simulink model "Adaptive_Event_send"  (R2023b)
settings: Solver=FixedStepDiscrete  StartTime=0.0  StopTime=50  RelTol=1e-3  EnableMultiTasking=on
undefined symbols (not defined in the file): gray, Rec, SDTV
libraries: visiontextngfix x4, visionconversions x3, visiongeotforms x2, autosarlibaprouting x1, raspberrypiAVlib x1
settings Model: Creator=seame-workstation09  LastModifiedBy=seame-workstation09
settings SolverCC: PositivePriorityOrder=on
settings OptimizationCC: DefaultParameterBehavior=Inlined  UseDivisionForNetSlopeComputation=on  GainParamInheritBuiltInType=on  UseFloatMulNetSlope=on  EnhancedBackFolding=on  PassReuseOutputArgsAs=Individual arguments  ZeroExternalMemoryAtStartup=off  ZeroInternalMemoryAtStartup=off  NoFixptDivByZeroProtection=on  EfficientFloat2IntCast=on  MaxStackSize=64  OptimizeBlockOrder=speed  DifferentSizesBufferReuse=on  OptimizationCustomize=off  EfficientTunableParamExpr=on
settings DebuggingCC: ParameterTunabilityLossMsg=error
settings HardwareCC: ProdBitPerLong=64  ProdLargestAtomicInteger=LongLong  ProdLargestAtomicFloat=Double  ProdLongLongMode=on  ProdHWDeviceType=ARM Compatible->ARM 64-bit (LP64)
settings SFSimCC: SimGenImportedTypeDefs=on  MATLABDynamicMemAlloc=off  SimTargetLang=C++
settings RTWCC: Description=AUTOSAR Adaptive  SystemTargetFile=autosar_adaptive.tlc  HardwareBoard=Embedded Coder Linux Docker Container  GenCodeOnly=on  TemplateMakefile=ert_default_tmf  Toolchain=AUTOSAR Adaptive Linux Executable  BuildConfiguration=Faster Runs  DataTypeReplacement=CDataTypesFixedWidth  TargetLang=C++
settings CodeAppCC: ForceParamTrailComments=on  IgnoreCustomStorageClasses=off  MaxIdLength=63  OperatorAnnotations=on  SimulinkDataObjDesc=on  SFDataObjDesc=on  CustomSymbolStrGlobalVar=rt$N$M  CustomSymbolStrType=$N$M  CustomSymbolStrFcn=$N$M$F  CustomSymbolStrMacro=$N$M  InsertBlockDesc=on
settings AUTOSARAdaptiveTargetCC: TargetFcnLib=ansi_tfl_table_tmw.mat  GenFloatMathFcnCalls=NOT IN USE  TargetLangStandard=C++11 (ISO)  CodeReplacementLibrary=None  UtilityFuncGeneration=Auto  MultiwordTypeDef=System defined  MultiwordLength=2048  DynamicStringBufferSize=256  GenerateFullHeader=on  InferredTypesCompatibility=off  GenerateSampleERTMain=off  GenerateTestInterfaces=off  ModelReferenceCompliant=on  ParMdlRefBuildCompliant=on  CompOptLevelCompliant=on  ConcurrentExecutionCompliant=on  IncludeMdlTerminateFcn=on  CombineOutputUpdateFcns=on  CombineSignalStateStructs=off  GroupInternalDataByFunction=off  SuppressErrorStatus=on  IncludeFileDelimiter=Auto  ERTCustomFileBanners=off  SupportAbsoluteTime=on  LogVarNameModifier=rt_  MatFileLogging=off  CodeInterfacePackaging=C++ class  PurelyIntegerCode=off  SupportNonFinite=off  SupportComplex=on  SupportContinuousTime=off  SupportNonInlinedSFcns=off  RemoveDisableFunc=off  RemoveResetFunc=on  SupportVariableSizeSignals=off  ParenthesesLevel=Nominal  CastingMode=Nominal  MATLABClassNameForMDSCustomization=Simulink.SoftwareTarget.TargetSpecificTriggerConfigurationBase  ModelStepFunctionPrototypeControlCompliant=off  CPPClassGenCompliant=on  AutosarCompliant=on  MDXCompliant=off  GRTInterface=off  GenerateAllocFcn=off  UseToolchainInfoCompliant=on  GenerateSharedConstants=on  CoderGroups=[]  AccessMethods=[]  LookupTableObjectStructAxisOrder=2,1,3,4,...  LUTObjectStructOrderExplicitValues=Size,Breakpoints,Table  LUTObjectStructOrderEvenSpacing=Size,Table,Breakpoints  ArrayLayout=Column-major  UnsupportedSFcnMsg=error  ERTHeaderFileRootName=$R$E  ERTSourceFileRootName=$R$E  ERTDataFileRootName=$R_data  OptimizeReductions=off  GenerateASAP2=off  DSAsUniqueAccess=off  ExtMode=on  ExtModeTransport=0  ExtModeStaticAlloc=off  ExtModeAutomaticAllocSize=on  ExtModeMaxTrigDuration=10  ExtModeStaticAllocSize=1000000  ExtModeTesting=off  ExtModeMexFile=ext_comm  ExtModeIntrfLevel=Level1  InlinedParameterPlacement=NonHierarchical  TargetOS=BareBoardExample  MultiInstanceErrorCode=Error  RootIOFormat=Structure reference  RTWCAPISignals=off  RTWCAPIParams=off  RTWCAPIStates=off  RTWCAPIRootIO=off  ERTSrcFileBannerTemplate=ert_code_template.cgt  ERTHdrFileBannerTemplate=ert_code_template.cgt  ERTDataSrcFileTemplate=ert_code_template.cgt  ERTDataHdrFileTemplate=ert_code_template.cgt  ERTCustomFileTemplate=example_file_process.tlc  EnableDataOwnership=off  SignalDisplayLevel=10  ParamTuneLevel=10  GlobalDataDefinition=Auto  DataDefinitionFile=global.c  GlobalDataReference=Auto  ERTFilePackagingFormat=Modular  RateTransitionBlockCode=Inline  DataReferenceFile=global.h  PreserveExpressionOrder=off  PreserveIfCondition=off  ConvertIfToSwitch=on  PreserveExternInFcnDecls=on  PreserveStaticInFcnDecls=on  SuppressUnreachableDefaultCases=on  EnableSignedLeftShifts=on  EnableSignedRightShifts=on  ImplementImageWithCVMat=off  IndentStyle=K&R  IndentSize=2  NewlineStyle=Default  MaxLineWidth=80  EnableUserReplacementTypes=off  MaxIdInt64=INT64_MAX  MinIdInt64=INT64_MIN  MaxIdUint64=UINT64_MAX  MaxIdInt32=INT32_MAX  MinIdInt32=INT32_MIN  MaxIdUint32=UINT32_MAX  MaxIdInt16=INT16_MAX  MinIdInt16=INT16_MIN  MaxIdUint16=UINT16_MAX  MaxIdInt8=INT8_MAX  MinIdInt8=INT8_MIN  MaxIdUint8=UINT8_MAX  BooleanTrueId=true  BooleanFalseId=false  MemSecPackage=--- None ---  MemSecDataConstants=Default  MemSecDataIO=Default  MemSecDataInternal=Default  MemSecDataParameters=Default  MemSecFuncInitTerm=Default  MemSecFuncExecute=Default  MemSecFuncSharedUtil=Default  GroupConstants=Default  GroupRootInputs=Default  GroupRootOutputs=Default  GroupInternal=Default  GroupParameters=Default  GroupDataTransfer=Default  GroupSharedLocalDataStores=Default  GroupInstanceSpecificParameters=Default  GroupModelData=Default  ArrayContainerType=std::array  AutosarSchemaVersion=R21-11  AutosarMaxShortNameLength=128  AdaptiveAutosarXCPServerTransportLayer=XCPOnTCPIP  AdaptiveAutosarXCPServerTCPIPAddress=192.168.86.20  AdaptiveAutosarXCPServerPort=22  AdaptiveAutosarXCPServerVerbosity=off  AdaptiveAutosarUseCustomXCPServer=off

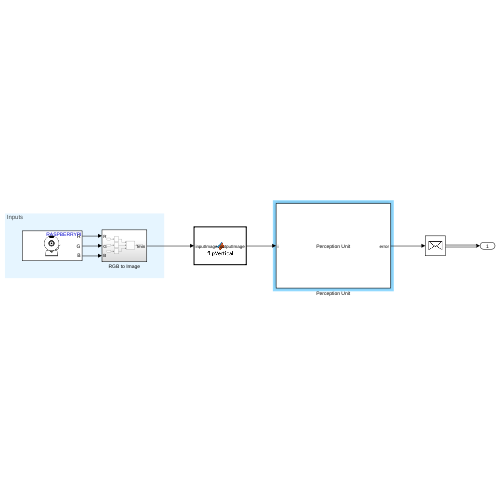
[thumbnail: Simulink's stored preview of the top-level diagram]
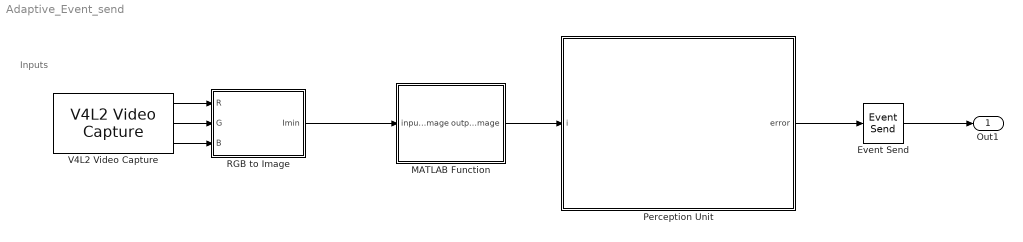
== system Adaptive_Event_send ==
  note: Inputs
  Event Send : autosarlibaprouting/Event Send
  MATLAB Function : MATLAB Function  TreatAsAtomicUnit=on
  Perception Unit : Subsystem  Description=Perception Unit
      mask Display: disp('Perception Unit');
  RGB to Image : Subsystem
  V4L2 Video Capture : raspberrypiAVlib/V4L2 Video Capture  DeviceName=/dev/video0  Resolution=640x480  CustomResolution=[2592,1944]  PixelFormat=RGB  SampleTime=0.1  pixelOrder=planar  simOutput=Colorbars  imSizeSelection=320x240  imSize=[640, 480]  roi=[0, 0, 640, 480]  m_devName='/dev/video0'  blockPlatform=LINUX  HorizontalFlip=off  VerticalFlip=off  Brightness=0.5  Saturation=0.5  Contrast=0.5  Sharpness=0.5  CameraPan=0  CameraTilt=0  CameraZoom=0.5  EnableManualFocus=on  ManualFocus=0.5
  Out1 : Outport
  wires:
  V4L2 Video Capture/1 -> RGB to Image/1(R)
  V4L2 Video Capture/2 -> RGB to Image/2(G)
  V4L2 Video Capture/3 -> RGB to Image/3(B)
  RGB to Image/1(Imin) -> MATLAB Function/1(inputImage)
  MATLAB Function/1(outputImage) -> Perception Unit/1(i)
  Perception Unit/1(error) -> Event Send/1
  Event Send/1 -> Out1/1

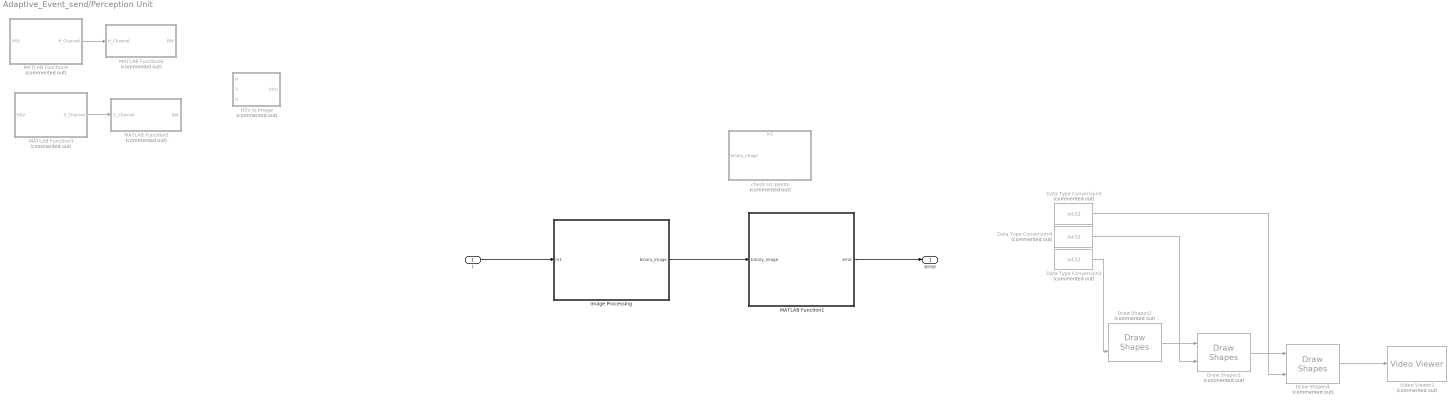
== system Adaptive_Event_send/Perception Unit ==
  i : Inport
  Data Type Conversion3 : DataTypeConversion  Commented=on  OutDataTypeStr=int32  SaturateOnIntegerOverflow=off  RndMeth=Floor
  Data Type Conversion4 : DataTypeConversion  Commented=on  OutDataTypeStr=int32  SaturateOnIntegerOverflow=off  RndMeth=Floor
  Data Type Conversion5 : DataTypeConversion  Commented=on  OutDataTypeStr=int32  SaturateOnIntegerOverflow=off  RndMeth=Floor
  Draw Shapes2 : visiontextngfix/Draw Shapes  Commented=on  shape=Rectangles  fill=off  lineWidth=1  fillClrSource=Specify via dialog  display=White  intensity=200  color=[0 255 0]  opacity=0.6  viewport=Entire image  antialiasing=off  inType=Obsolete  imagePorts=One multidimensional signal  roundingMode=Floor  overflowMode=off  memoryMode=Specify word length  memoryWordLength=16  prodOutputMode=Binary point scaling  prodOutputWordLength=32  prodOutputFracLength=14  memoryFracLength=15
  Draw Shapes3 : visiontextngfix/Draw Shapes  Commented=on  shape=Circles  fill=on  lineWidth=1  fillClrSource=Specify via dialog  display=Black  intensity=200  color=[0 255 0]  opacity=0.8  viewport=Entire image  antialiasing=off  inType=Obsolete  imagePorts=One multidimensional signal  roundingMode=Floor  overflowMode=off  memoryMode=Specify word length  memoryWordLength=16  prodOutputMode=Binary point scaling  prodOutputWordLength=32  prodOutputFracLength=14  memoryFracLength=15
  Draw Shapes4 : visiontextngfix/Draw Shapes  Commented=on  shape=Lines  fill=off  lineWidth=4  fillClrSource=Specify via dialog  display=Black  intensity=200  color=[255 0 0]  opacity=0.6  viewport=Entire image  antialiasing=off  inType=Obsolete  imagePorts=One multidimensional signal  roundingMode=Floor  overflowMode=off  memoryMode=Specify word length  memoryWordLength=16  prodOutputMode=Binary point scaling  prodOutputWordLength=32  prodOutputFracLength=14  memoryFracLength=14
  HSV to Image : Subsystem  Commented=on
  Image Processing : Subsystem
  MATLAB Function1 : MATLAB Function  TreatAsAtomicUnit=on
  MATLAB Function3 : MATLAB Function  Commented=on  TreatAsAtomicUnit=on
  MATLAB Function4 : MATLAB Function  Commented=on  TreatAsAtomicUnit=on
  MATLAB Function5 : MATLAB Function  Commented=on  TreatAsAtomicUnit=on
  MATLAB Function6 : MATLAB Function  Commented=on  TreatAsAtomicUnit=on
  Video Viewer2 : VideoViewer  Commented=on  colormapValue=gray(256)  FigPos=[498 952 1161 594]
  check src points : Subsystem  Commented=on
      settings: PortSchema="{\"entries\":[{\"content\":{\"sides\":[{\"content\":{\"connectorIds\":[\"In1\"]},\"type\":\"ConnectorPlacement.EquallySpacedRectSide\",\"uuid\":\"f9a6de61-1898-4465-aab1-5f75a88d6bc5\"},{\"content\":{\"side\":\"RIGHT\"},\"type\":\"ConnectorPlacement.EquallySpacedRectSide\",\"uuid\":\"22a87883-a793-424b-ac6e-07d139e6a826\"},{\"content\":{\"connectorIds\":[\"In2\"],\"side\":\"TOP\"},\"type\":\"ConnectorPlacement.EquallySpacedRectSide\",\"uuid\":\"93f3f8a5-f2dd-45b6-b00d-0d3a0a24e380\"}]},\"type\":\"ConnectorPlacement.EquallySpacedConnector\",\"uuid\":\"35037751-f37a-49b1-b87d-24865a03c27c\"}],\"packageUris\":[\"http://schema.mathworks.com/mf0/Connector/R2020b\"],\"version\":\"1.0\"}"
  error : Outport  VectorParamsAs1DForOutWhenUnconnected=off
  wires:
  MATLAB Function4/1(H_Channel) -> MATLAB Function6/1(H_Channel)
  MATLAB Function3/1(S_Channel) -> MATLAB Function5/1(S_Channel)
  i/1 -> Image Processing/1(In1)
  Image Processing/1(binary_image) -> MATLAB Function1/1(binary_image)
  Data Type Conversion3/1 -> Draw Shapes2/2
  Data Type Conversion4/1 -> Draw Shapes3/2
  Draw Shapes2/1 -> Draw Shapes3/1
  Draw Shapes3/1 -> Draw Shapes4/1
  Data Type Conversion5/1 -> Draw Shapes4/2
  MATLAB Function1/1(error) -> error/1
  Draw Shapes4/1 -> Video Viewer2/1

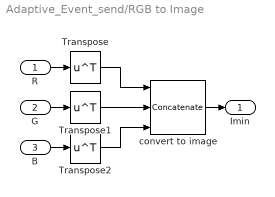
== system Adaptive_Event_send/RGB to Image ==
  R : Inport
  G : Inport  Port=2
  B : Inport  Port=3
  Transpose : Math  Operator=transpose
  Transpose1 : Math  Operator=transpose
  Transpose2 : Math  Operator=transpose
  convert to image : Concatenate  NumInputs=3  Mode=Multidimensional array  ConcatenateDimension=3
  Imin : Outport
  wires:
  R/1 -> Transpose/1
  G/1 -> Transpose1/1
  Transpose/1 -> convert to image/1
  Transpose1/1 -> convert to image/2
  B/1 -> Transpose2/1
  Transpose2/1 -> convert to image/3
  convert to image/1 -> Imin/1

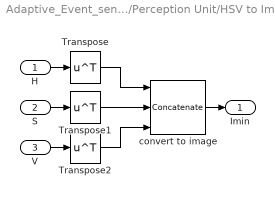
== system Adaptive_Event_send/Perception Unit/HSV to Image ==
  H : Inport
  S : Inport  Port=2
  V : Inport  Port=3
  Transpose : Math  Operator=transpose
  Transpose1 : Math  Operator=transpose
  Transpose2 : Math  Operator=transpose
  convert to image : Concatenate  NumInputs=3  Mode=Multidimensional array  ConcatenateDimension=3
  Imin : Outport
  wires:
  H/1 -> Transpose/1
  S/1 -> Transpose1/1
  Transpose/1 -> convert to image/1
  Transpose1/1 -> convert to image/2
  V/1 -> Transpose2/1
  Transpose2/1 -> convert to image/3
  convert to image/1 -> Imin/1

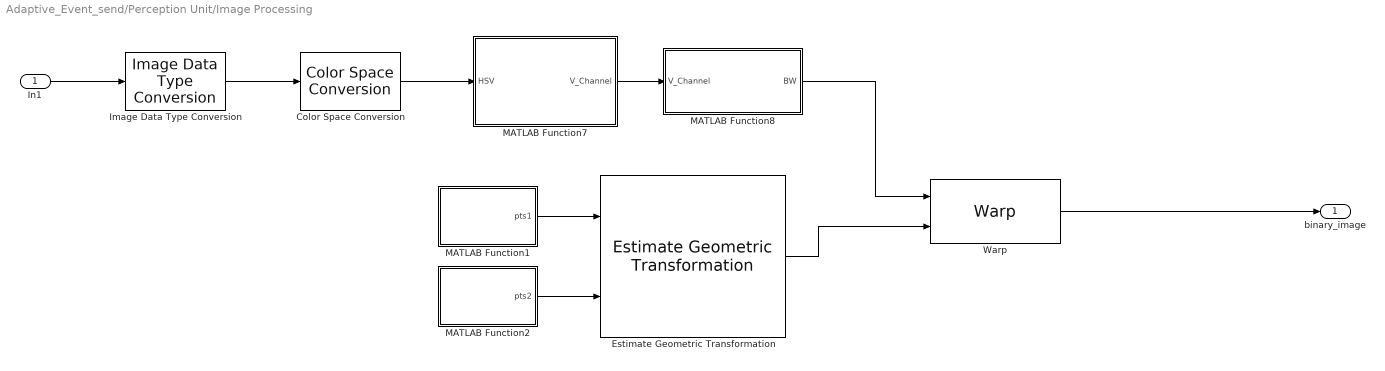
== system Adaptive_Event_send/Perception Unit/Image Processing ==
  In1 : Inport
  Color Space Conversion : visionconversions/Color Space  Conversion  conversion=Obsolete  conversionActive=R'G'B' to HSV  wp_str=D65  rec=Rec. 601 (SDTV)  sys=1125/60/2:1  imagePorts=One multidimensional signal
  Estimate Geometric Transformation : visiongeotforms/Estimate Geometric Transformation  tformType=Projective  isRandomSampling=on  algMethod=Random Sample Consensus (RANSAC)  distanceAlg=2.5  distanceGeo=2.5  numMethod=Specified value  sampleNum=500  desiredConfidence=99  maxSampleNum=1000  isStopSampling=off  percentStop=75  isRefineTForm=off  isReleaseMode=on  isOutputInlier=off  outDT4IntInput=Obsolete10a  outDT4IntInputActive=Single  isVarSizeAllowed=on
  Image Data Type Conversion : visionconversions/Image Data Type Conversion  outDT=double  isSigned=on  wordLen=16  numFracBits=0
  MATLAB Function1 : MATLAB Function  TreatAsAtomicUnit=on
  MATLAB Function2 : MATLAB Function  TreatAsAtomicUnit=on
  MATLAB Function7 : MATLAB Function  TreatAsAtomicUnit=on
  MATLAB Function8 : MATLAB Function  TreatAsAtomicUnit=on
  Warp : visiongeotforms/Warp  TransformMatrixSource=Input port  TransformMatrix=eye( 3 )  InterpolationMethod=Bilinear  BackgroundFillValue=0  OutputImagePositionSource=Same as input image  OutputImagePosition=[ 1, 1, 512, 512 ]  ROIInputPort=off  ROIValidityOutputPort=off  SimulateUsing=Interpreted execution
  binary_image : Outport
  wires:
  MATLAB Function8/1(BW) -> Warp/1
  Image Data Type Conversion/1 -> Color Space Conversion/1
  MATLAB Function1/1(pts1) -> Estimate Geometric Transformation/1
  MATLAB Function7/1(V_Channel) -> MATLAB Function8/1(V_Channel)
  MATLAB Function2/1(pts2) -> Estimate Geometric Transformation/2
  Estimate Geometric Transformation/1 -> Warp/2
  Color Space Conversion/1 -> MATLAB Function7/1(HSV)
  Warp/1 -> binary_image/1
  In1/1 -> Image Data Type Conversion/1

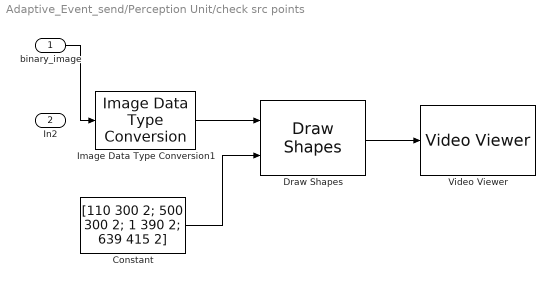
== system Adaptive_Event_send/Perception Unit/check src points ==
  binary_image : Inport
  In2 : Inport  Port=2
  Constant : Constant  Value=[110 300 2; 500 300 2; 1 390 2; 639 415 2]
  Draw Shapes : visiontextngfix/Draw Shapes  shape=Circles  fill=on  lineWidth=1  fillClrSource=Specify via dialog  display=White  intensity=200  color=crea2  opacity=0.8  viewport=Entire image  antialiasing=off  inType=Obsolete  imagePorts=One multidimensional signal  roundingMode=Floor  overflowMode=off  memoryMode=Specify word length  memoryWordLength=16  prodOutputMode=Binary point scaling  prodOutputWordLength=32  prodOutputFracLength=14  memoryFracLength=15
  Image Data Type Conversion1 : visionconversions/Image Data Type Conversion  outDT=double  isSigned=on  wordLen=16  numFracBits=0
  Video Viewer : VideoViewer  colormapValue=gray(256)  FigPos=[184 922 1283 663]
  wires:
  Constant/1 -> Draw Shapes/2
  binary_image/1 -> Image Data Type Conversion1/1
  Image Data Type Conversion1/1 -> Draw Shapes/1
  Draw Shapes/1 -> Video Viewer/1

== matlab function Adaptive_Event_send/Perception Unit/Image Processing/MATLAB Function1 ==
  data: pts1 output
function pts1 = getpts1()

pts1 = [110 300
        500 300
        1 390
        639 415];

end

== matlab function Adaptive_Event_send/Perception Unit/MATLAB Function3 ==
  data: S_Channel output; HSV input
function S_Channel = get_SChannel(HSV)

S_Channel = HSV(:,:,2);

end

== matlab function Adaptive_Event_send/Perception Unit/Image Processing/MATLAB Function2 ==
  data: pts2 output
function pts2 = getpts2()

pts2 = [40 300
        600 300
        40 480
        600 480];

end

== matlab function Adaptive_Event_send/Perception Unit/MATLAB Function5 ==
  data: BW output; S_Channel input
function BW = mask(S_Channel)
S_th = 0.5;

BW = S_Channel < S_th;

end

== matlab function Adaptive_Event_send/Perception Unit/Image Processing/MATLAB Function7 ==
  data: V_Channel output; HSV input
function V_Channel = get_VChannel(HSV)

V_Channel = HSV(:,:,3);

end

== matlab function Adaptive_Event_send/Perception Unit/Image Processing/MATLAB Function8 ==
  data: BW output; V_Channel input
function BW = mask(V_Channel)
V_th = 0.5;

BW = V_Channel > V_th;

end

== matlab function Adaptive_Event_send/Perception Unit/MATLAB Function6 ==
  data: BW output; H_Channel input
function BW = mask(H_Channel)
H_th = 0.45;

BW = H_Channel > H_th;

end

== matlab function Adaptive_Event_send/Perception Unit/MATLAB Function4 ==
  data: H_Channel output; HSV input
function H_Channel = get_HChannel(HSV)

H_Channel = HSV(:,:,1);

end

== matlab function Adaptive_Event_send/MATLAB Function ==
  data: inputImage input; outputImage output
function outputImage = flipVertical(inputImage)

    tempImage = flipud(inputImage);
    outputImage = fliplr(tempImage)
end

== matlab function Adaptive_Event_send/Perception Unit/MATLAB Function1 ==
  data: binary_image input; error output
% function error   = Lane_Detection(binary_image)
function error   = Lane_Detection(binary_image)

h = size(binary_image,1);
w = size(binary_image,2);

mid_w = w / 2;
x_location = 320;

nwindows = 20; % 윈도우 개수 (number of windows)

window_hight = h/nwindows; % 윈도우별 높이(고정) (height of each window)


margin = 40; % 윈도우 너비 결정 (margin determine width of window)
minpix = 30;

max_points = 100000; % 정적 배열 할당 위한 행(point 개수) 지정 (maximum size of row for static array)

% 슬라이딩 윈도우를 통해 탐색된 차선 픽셀들 담을 list (list for storing pixels which are found from sliding window algorithm)

left_lane_index = zeros(max_points, 2);
right_lane_index = zeros(max_points, 2);

[nonzeroy, nonzerox] = find(binary_image); % 흰색 픽셀(차선)의 x, y 좌표 찾음 (found pixel's location which has '1' value(which means white))

% static 
count_left = 0; % 몇개의 행(points)이 사용됐는지 추적 위한 count (to count how many points are stored)
count_right = 0;

rectangle_points = zeros(2 * nwindows + 2,4); % 각 윈도우들의 경계를 저장하기 위한 행렬, 0으로 초기화, 윈도우 개수*2(왼쪽, 오른쪽), 4개의 열(x, y, w, h) (setting array for each widow's boundary)

% 좌측, 우측 first 윈도우 사이즈 (size of window)
win_y_low = h - window_hight;
win_y_high = h;

win_xleft_low = 0;
win_xleft_high = 160;
win_xright_low = 480;
win_xright_high = 640;


rectangle_points(41,:) = [win_xleft_low win_y_low 4*margin window_hight]; % [x, y, w, h]
rectangle_points(42,:) = [win_xright_low win_y_low 4*margin window_hight];


good_leftx_indexs = nonzerox((nonzeroy >= win_y_low) & (nonzeroy < win_y_high) & (nonzerox >= win_xleft_low) &  (nonzerox < win_xleft_high)); 
good_lefty_indexs = nonzeroy((nonzeroy >= win_y_low) & (nonzeroy < win_y_high) & (nonzerox >= win_xleft_low) &  (nonzerox < win_xleft_high));

good_rightx_indexs = nonzerox((nonzeroy >= win_y_low) & (nonzeroy < win_y_high) & (nonzerox >= win_xright_low) &  (nonzerox < win_xright_high));
good_righty_indexs = nonzeroy((nonzeroy >= win_y_low) & (nonzeroy < win_y_high) & (nonzerox >= win_xright_low) &  (nonzerox < win_xright_high));

% 왼쪽차선, 오른쪽차선 인덱스 list에 추출된 픽셀 인덱스를 각각 추가 (store indeox found from
% current window to array)
% method1: static 
for j = count_left+1:numel(good_leftx_indexs)
    left_lane_index(j, :) = [good_leftx_indexs(j), good_lefty_indexs(j)];
    count_left = count_left + 1;
end

for j = count_right+1:numel(good_rightx_indexs)
    right_lane_index(j, :) = [good_rightx_indexs(j), good_righty_indexs(j)];
    count_right = count_right + 1;
end


if(numel(good_rightx_indexs) > 30)
    line_flag = 1;
    x_current = mean(good_rightx_indexs);
    y_current = max(good_righty_indexs);
else
    line_flag = 2;
    x_current = mean(good_leftx_indexs);
    y_current = max(good_lefty_indexs);
end

mean_points = [x_current y_current 2];

% static 
count_left = 0; % 몇개의 행(points)이 사용됐는지 추적 위한 count (to count how many points are stored)
count_right = 0;




for i = 1:nwindows
    if (line_flag == 1)
        win_y_low = y_current - (i+1)*window_hight;
        win_y_high = y_current - i*window_hight;
        win_x_low = x_current - margin;
        win_x_high = x_current + margin;

        rectangle_points(i,:) = [win_x_low win_y_low 2*margin window_hight]; % right [x, y, w, h]
        rectangle_points(nwindows+i,:) = [win_x_low-520 win_y_low 2*margin window_hight]; % left

        good_rightx_indexs = nonzerox((nonzeroy >= win_y_low) & (nonzeroy < win_y_high) & (nonzerox >= win_x_low) &  (nonzerox < win_x_high));
        good_righty_indexs = nonzeroy((nonzeroy >= win_y_low) & (nonzeroy < win_y_high) & (nonzerox >= win_x_low) &  (nonzerox < win_x_high));

        if(numel(good_rightx_indexs) > minpix)
            x_current = mean(good_rightx_indexs);
        end

        if((win_y_low > 300) && (win_y_low < 340))
            x_location = x_current - 260;
        end

        for j = count_right+1:numel(good_rightx_indexs)
            right_lane_index(j, :) = [good_rightx_indexs(j), good_righty_indexs(j)];
            left_lane_index(j, :) = [good_rightx_indexs(j)-520, good_righty_indexs(j)];
            count_right = count_right + 1;
        end

    end

    if (line_flag == 2)
        win_y_low = y_current - (i+1)*window_hight;
        win_y_high = y_current - i*window_hight;
        win_x_low = x_current - margin;
        win_x_high = x_current + margin;

        rectangle_points(i,:) = [win_x_low win_y_low 2*margin window_hight]; % left [x, y, w, h]
        rectangle_points(nwindows+i,:) = [win_x_low+520 win_y_low 2*margin window_hight]; % right

        good_leftx_indexs = nonzerox((nonzeroy >= win_y_low) & (nonzeroy < win_y_high) & (nonzerox >= win_x_low) &  (nonzerox < win_x_high));
        good_lefty_indexs = nonzeroy((nonzeroy >= win_y_low) & (nonzeroy < win_y_high) & (nonzerox >= win_x_low) &  (nonzerox < win_x_high));

        if(numel(good_leftx_indexs) > minpix)
            x_current = mean(good_leftx_indexs);
        end
        
        if((win_y_low > 300) && (win_y_low < 340))
            x_location = x_current + 260;
        end

        for j = count_left+1:numel(good_leftx_indexs)
            left_lane_index(j, :) = [good_leftx_indexs(j), good_lefty_indexs(j)];
            right_lane_index(j, :) = [good_leftx_indexs(j)+520, good_lefty_indexs(j)];
            count_left = count_left + 1;
        end

    end

    error = mid_w - x_location;
end
